simulink model "dynamicANN"  (R2019b)
settings: Solver=VariableStepAuto  StartTime=0.0  StopTime=5  RelTol=1e-3
values from neighbouring files (symbols this model uses):
  a = 87.548e-3    (= 0.087548)    [main.m]
  b = 132.452e-3    (= 0.132452)    [main.m]
  d = 22.452e-3    (= 0.022452)    [main.m]
  delta = [dX 0 0 0; -dX 0 0 0; 0 dXdot 0 0; 0 -dXdot 0 0; 0 0 dY 0; 0 0 -dY 0; 0 0 0 dYdot; 0 0 0 -dYdot]    [dyn_coeff.m]    (also in main.m = 2.5e-05)
  F1 = mass*g-F2    (= 22.4020462598)    [main.m]
  F2 = a*mass*g/(a+b)    (= 14.8072837402)    [main.m]
  g = 9.8    [EOM.m]    (also in main.m = 9.81)
  Jd = 0.047331604    [main.m]
  Jp = 0.00075    [main.m]
  Kps = (Vmax-Vmin)/(Hmax-Hmin)    (= 1666.66666667)    [main.m]
  Ksv = 30    [main.m]
  mass = 3.793    [main.m]
  omega = operational_parameters(1)*2*pi/60    [CalculateLoadCapacity.m]    (also in main.m = 146.607657168)
  s = 30e-3    (= 0.03)    [main.m]    (also in nntrainingsetgen.m = size(XC))
  tau = 0.12    [main.m]
  taus = 0.00125    [main.m]
  Ts = 1/fs    (= 0.001)    [main.m]
libraries: neural x424, simulink x2
(part 1 of 10)
settings Model: Creator=Alexander  LastModifiedBy=Alexander

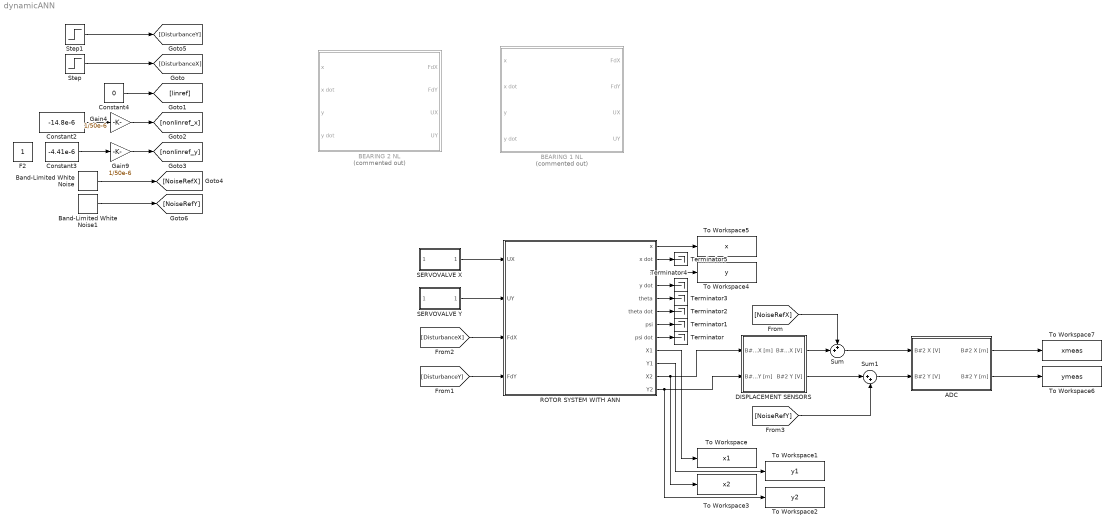
== system dynamicANN ==
  ADC : Subsystem
  BEARING 1 NL : Subsystem  Commented=on
  BEARING 2 NL : Subsystem  Commented=on
  Band-Limited White Noise : simulink/Sources/Band-Limited White Noise  Cov=n_pow  Ts=Ts  seed=[23341]
  Band-Limited White Noise1 : simulink/Sources/Band-Limited White Noise  Cov=n_pow  Ts=1.1*Ts  seed=[23341]
  Constant2 : Constant  Value=-14.8e-6
  Constant3 : Constant  Value=-4.41e-6
  Constant4 : Constant  Value=0
  DISPLACEMENT SENSORS : Subsystem
  Gain4 : Gain  Gain=1/50e-6
  Gain9 : Gain  Gain=1/50e-6
  ROTOR SYSTEM WITH ANN : Subsystem
  SERVOVALVE X : Subsystem
  SERVOVALVE Y : Subsystem
  Step : Step  After=-15  SampleTime=0
  Step1 : Step  After=-15  SampleTime=0
  Sum : Sum  Inputs=++|
  Sum1 : Sum  Inputs=|++
  Terminator{,1..5} (6 alike) : Terminator
  To Workspace : ToWorkspace  VariableName=x1  SampleTime=-1
      settings: Save2DSignal=2-D array (concatenate along first dimension)
  To Workspace1 : ToWorkspace  VariableName=y1  SampleTime=-1
      settings: Save2DSignal=2-D array (concatenate along first dimension)
  To Workspace2 : ToWorkspace  VariableName=y2  SampleTime=-1
      settings: Save2DSignal=2-D array (concatenate along first dimension)
  To Workspace3 : ToWorkspace  VariableName=x2  SampleTime=-1
      settings: Save2DSignal=2-D array (concatenate along first dimension)
  To Workspace4 : ToWorkspace  VariableName=y  SampleTime=-1
      settings: Save2DSignal=2-D array (concatenate along first dimension)
  To Workspace5 : ToWorkspace  VariableName=x  SampleTime=-1
      settings: Save2DSignal=2-D array (concatenate along first dimension)
  To Workspace6 : ToWorkspace  VariableName=ymeas  SampleTime=-1
      settings: Save2DSignal=2-D array (concatenate along first dimension)
  To Workspace7 : ToWorkspace  VariableName=xmeas  SampleTime=-1
      settings: Save2DSignal=2-D array (concatenate along first dimension)
  F2 : Constant  IOType=siggen
  wires:
  ROTOR SYSTEM WITH ANN/10(Y1) -> To Workspace1/1
  ROTOR SYSTEM WITH ANN/9(X1) -> To Workspace/1
  ROTOR SYSTEM WITH ANN/8(psi dot) -> Terminator/1
  ROTOR SYSTEM WITH ANN/6("theta dot ") -> Terminator2/1
  ROTOR SYSTEM WITH ANN/7(psi) -> Terminator1/1
  ROTOR SYSTEM WITH ANN/4(y dot) -> Terminator4/1
  ROTOR SYSTEM WITH ANN/5(theta) -> Terminator3/1
  ROTOR SYSTEM WITH ANN/2(x dot) -> Terminator5/1
  ROTOR SYSTEM WITH ANN/3(y) -> To Workspace4/1
  ROTOR SYSTEM WITH ANN/1("x ") -> To Workspace5/1
  SERVOVALVE Y/1(Uf [F]) -> ROTOR SYSTEM WITH ANN/2(UY)
  SERVOVALVE X/1(Uf [F]) -> ROTOR SYSTEM WITH ANN/1(UX)
  Constant3/1 -> Gain9/1
  Step1/1 -> [DisturbanceY]
  Gain9/1 -> [nonlinref_y]
  Constant2/1 -> Gain4/1
  Constant4/1 -> [linref]
  Step/1 -> [DisturbanceX]
  Gain4/1 -> [nonlinref_x]
  [DisturbanceY] -> ROTOR SYSTEM WITH ANN/4(FdY)
  [DisturbanceX] -> ROTOR SYSTEM WITH ANN/3(FdX)
  Band-Limited White Noise/1 -> [NoiseRefX]
  Band-Limited White Noise1/1 -> [NoiseRefY]
  [NoiseRefY] -> Sum1/2
  Sum/1 -> ADC/1(B#2 X [V])
  Sum1/1 -> ADC/2(B#2 Y [V])
  ADC/2(B#2 Y [m]) -> To Workspace6/1
  ADC/1(B#2 X [m]) -> To Workspace7/1
  ROTOR SYSTEM WITH ANN/12(Y2) -> To Workspace2/1, DISPLACEMENT SENSORS/2(B#2 Y [m])
  ROTOR SYSTEM WITH ANN/11("X2 ") -> To Workspace3/1, DISPLACEMENT SENSORS/1(B#2 X [m])
  DISPLACEMENT SENSORS/1(B#2 X [V]) -> Sum/2
  DISPLACEMENT SENSORS/2(B#2 Y [V]) -> Sum1/1
  [NoiseRefX] -> Sum/1

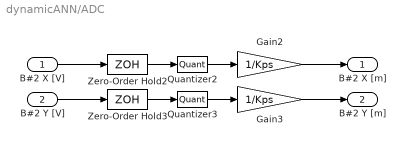
== system dynamicANN/ADC ==
  B#2 X [V] : Inport
  B#2 Y [V] : Inport  Port=2
  Gain2 : Gain  Gain=1/Kps
  Gain3 : Gain  Gain=1/Kps
  Quantizer2 : Quantizer  QuantizationInterval=0.000152587890625
  Quantizer3 : Quantizer  QuantizationInterval=0.000152587890625
  Zero-Order Hold2 : ZeroOrderHold  SampleTime=Ts
  Zero-Order Hold3 : ZeroOrderHold  SampleTime=Ts
  B#2 X [m] : Outport
  B#2 Y [m] : Outport  Port=2
  wires:
  Quantizer2/1 -> Gain2/1
  Quantizer3/1 -> Gain3/1
  B#2 X [V]/1 -> Zero-Order Hold2/1
  Gain2/1 -> B#2 X [m]/1
  Zero-Order Hold2/1 -> Quantizer2/1
  Gain3/1 -> B#2 Y [m]/1
  Zero-Order Hold3/1 -> Quantizer3/1
  B#2 Y [V]/1 -> Zero-Order Hold3/1

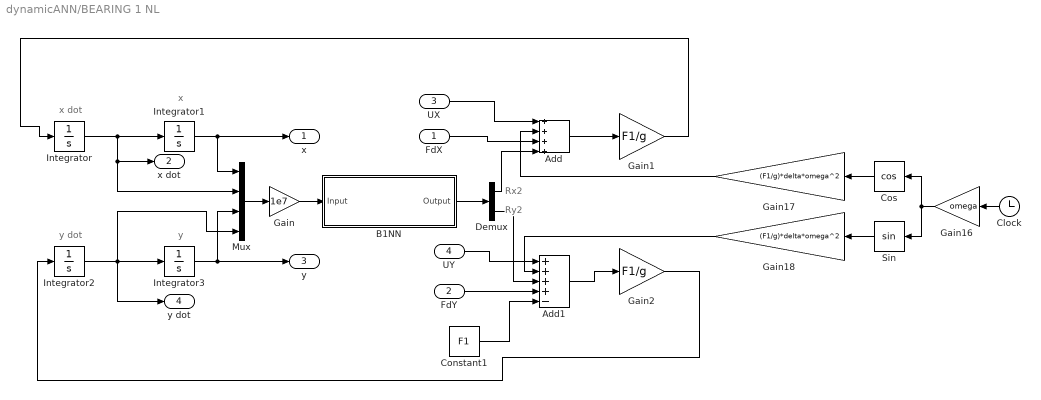
== system dynamicANN/BEARING 1 NL ==
  note: y
  note: x dot
  note: y dot
  note: Rx2
  note: Ry2
  note: x
  FdX : Inport
  FdY : Inport  Port=2
  UX : Inport  Port=3
  UY : Inport  Port=4
  Add : Sum  Inputs=++++
  Add1 : Sum  Inputs=++++-
  B1NN : Subsystem
      mask help: Feed-Forward Neural Network
      mask Display: fprintf('BEARIN #1 NN');port_label('input',1,' X');port_label('output',1,'F');
  Clock : Clock
  Constant1 : Constant  Value=F1
  Cos : Trigonometry  Operator=cos
  Demux : Demux  Outputs=2
  Gain : Gain  Gain=1e7
  Gain1 : Gain  Gain=F1/g
  Gain16 : Gain  Gain=omega
  Gain17 : Gain  Gain=(F1/g)*delta*omega^2
  Gain18 : Gain  Gain=(F1/g)*delta*omega^2
  Gain2 : Gain  Gain=F1/g
  Integrator{,1..3} (4 alike) : Integrator
  Mux : Mux
  Sin : Trigonometry
  x : Outport
  "x dot " : Outport  Port=2
  y : Outport  Port=3
  y dot : Outport  Port=4
  wires:
  Mux/1 -> Gain/1
  B1NN/1(Output) -> Demux/1
  Gain/1 -> B1NN/1(Input)
  Integrator1/1 -> x/1, Mux/1
  Integrator2/1 -> y dot/1, Mux/4, Integrator3/1
  Integrator/1 -> "x dot "/1, Mux/2, Integrator1/1
  Integrator3/1 -> y/1, Mux/3
  Clock/1 -> Gain16/1
  Sin/1 -> Gain18/1
  Cos/1 -> Gain17/1
  Gain2/1 -> Integrator2/1
  Add/1 -> Gain1/1
  Gain16/1 -> Sin/1, Cos/1
  Add1/1 -> Gain2/1
  Gain17/1 -> Add/2
  Gain18/1 -> Add1/2
  Gain1/1 -> Integrator/1
  FdX/1 -> Add/3
  Demux/1 -> Add/4
  FdY/1 -> Add1/4
  Constant1/1 -> Add1/5
  UX/1 -> Add/1
  Demux/2 -> Add1/3
  UY/1 -> Add1/1

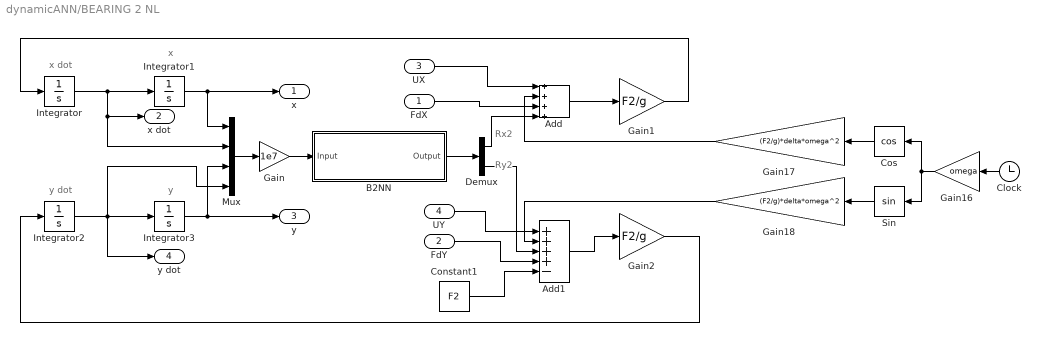
== system dynamicANN/BEARING 2 NL ==
  note: x
  note: x dot
  note: y
  note: y dot
  note: Ry2
  note: Rx2
  FdX : Inport
  FdY : Inport  Port=2
  UX : Inport  Port=3
  UY : Inport  Port=4
  Add : Sum  Inputs=++++
  Add1 : Sum  Inputs=++++-
  B2NN : Subsystem
      mask help: Feed-Forward Neural Network
      mask Display: fprintf('BEARING #2 NN');port_label('input',1,' X');port_label('output',1,'F');
  Clock : Clock
  Constant1 : Constant  Value=F2
  Cos : Trigonometry  Operator=cos
  Demux : Demux  Outputs=2
  Gain : Gain  Gain=1e7
  Gain1 : Gain  Gain=F2/g
  Gain16 : Gain  Gain=omega
  Gain17 : Gain  Gain=(F2/g)*delta*omega^2
  Gain18 : Gain  Gain=(F2/g)*delta*omega^2
  Gain2 : Gain  Gain=F2/g
  Integrator{,1..3} (4 alike) : Integrator
  Mux : Mux
  Sin : Trigonometry
  x : Outport
  "x dot " : Outport  Port=2
  y : Outport  Port=3
  y dot : Outport  Port=4
  wires:
  Add1/1 -> Gain2/1
  Gain1/1 -> Integrator/1
  FdY/1 -> Add1/4
  Integrator/1 -> "x dot "/1, Mux/2, Integrator1/1
  Integrator1/1 -> x/1, Mux/1
  Integrator2/1 -> y dot/1, Mux/4, Integrator3/1
  Add/1 -> Gain1/1
  Integrator3/1 -> y/1, Mux/3
  FdX/1 -> Add/3
  Mux/1 -> Gain/1
  Demux/2 -> Add1/3
  Gain/1 -> B2NN/1(Input)
  Demux/1 -> Add/4
  Gain2/1 -> Integrator2/1
  Constant1/1 -> Add1/5
  B2NN/1(Output) -> Demux/1
  Sin/1 -> Gain18/1
  Cos/1 -> Gain17/1
  Gain16/1 -> Sin/1, Cos/1
  Clock/1 -> Gain16/1
  Gain17/1 -> Add/2
  Gain18/1 -> Add1/2
  UX/1 -> Add/1
  UY/1 -> Add1/1

== system dynamicANN/DISPLACEMENT SENSORS ==
  B#2 X [m] : Inport
  B#2 Y [m] : Inport  Port=2
  Transfer Fcn2 : TransferFcn  Numerator=[Kps]  Denominator=[taus 1]
  Transfer Fcn3 : TransferFcn  Numerator=[Kps]  Denominator=[taus 1]
  B#2 X [V] : Outport
  B#2 Y [V] : Outport  Port=2
  wires:
  B#2 Y [m]/1 -> Transfer Fcn3/1
  B#2 X [m]/1 -> Transfer Fcn2/1
  Transfer Fcn2/1 -> B#2 X [V]/1
  Transfer Fcn3/1 -> B#2 Y [V]/1

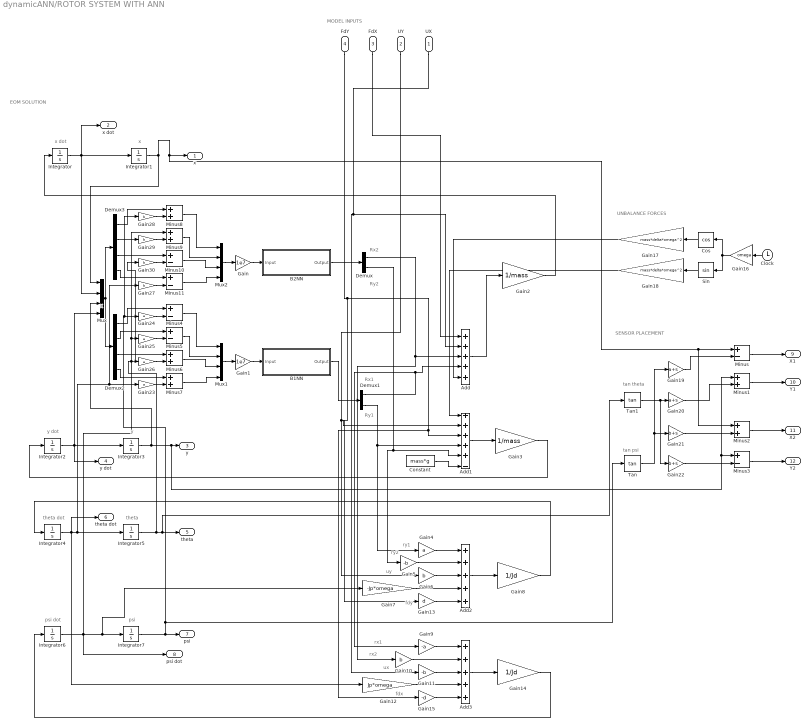
== system dynamicANN/ROTOR SYSTEM WITH ANN ==
  note: SENSOR PLACEMENT
  note: tan theta
  note: EOM SOLUTION
  note: MODEL INPUTS
  note: UNBALANCE FORCES
  note: fdx
  note: ux
  note: rx2
  note: rx1
  note: fdy
  note: uy
  note: ry2
  note: ry1
  note: Ry2
  note: Rx2
  note: X
  note: x dot
  note: x
  note: y
  note: y dot
  note: Ry1
  note: Rx1
  note: theta dot
  note: theta
  note: psi dot
  note: psi
  note: tan psi
  UX : Inport
  UY : Inport  Port=2
  FdX : Inport  Port=3
  FdY : Inport  Port=4
  Add : Sum  Inputs=+++++
  Add1 : Sum  Inputs=+++++-
  Add2 : Sum  Inputs=+++++
  Add3 : Sum  Inputs=+++++
  B1NN : Subsystem
      mask help: Feed-Forward Neural Network
      mask Display: fprintf('BEARIN #1 NN');port_label('input',1,' X');port_label('output',1,'F');
  B2NN : Subsystem
      mask help: Feed-Forward Neural Network
      mask Display: fprintf('BEARING #2 NN');port_label('input',1,' X');port_label('output',1,'F');
  Clock : Clock
  Constant : Constant  Value=mass*g
  Cos : Trigonometry  Operator=cos
  Demux : Demux  Outputs=2
  Demux1 : Demux  Outputs=2
  Demux2 : Demux
  Demux3 : Demux
  Gain : Gain  Gain=1e7
  Gain1 : Gain  Gain=1e7
  Gain{6,10,27..30} (6 alike) : Gain  Gain=b
  Gain11 : Gain  Gain=-b
  Gain12 : Gain  Gain=Jp*omega
  Gain13 : Gain  Gain=d
  Gain14 : Gain  Gain=1/Jd
  Gain15 : Gain  Gain=-d
  Gain16 : Gain  Gain=omega
  Gain17 : Gain  Gain=mass*delta*omega^2
  Gain18 : Gain  Gain=mass*delta*omega^2
  Gain19 : Gain  Gain=a+s
  Gain2 : Gain  Gain=1/mass
  Gain20 : Gain  Gain=a+s
  Gain21 : Gain  Gain=b+s
  Gain22 : Gain  Gain=b+s
  Gain{4,23..26} (5 alike) : Gain  Gain=a
  Gain3 : Gain  Gain=1/mass
  Gain5 : Gain  Gain=-b
  Gain7 : Gain  Gain=-Jp*omega
  Gain8 : Gain  Gain=1/Jd
  Gain9 : Gain  Gain=-a
  Integrator{,1..7} (8 alike) : Integrator
  Minus{,3..5,10..11} (6 alike) : Sum  Inputs=+-
  Minus{1..2,6..9} (6 alike) : Sum
  Mux : Mux
  Mux1 : Mux
  Mux2 : Mux
  Sin : Trigonometry
  Tan : Trigonometry  Operator=tan
  Tan1 : Trigonometry  Operator=tan
  "x " : Outport
  x dot : Outport  Port=2
  y : Outport  Port=3
  y dot : Outport  Port=4
  theta : Outport  Port=5
  "theta dot " : Outport  Port=6
  psi : Outport  Port=7
  psi dot : Outport  Port=8
  X1 : Outport  Port=9
  Y1 : Outport  Port=10
  "X2 " : Outport  Port=11
  Y2 : Outport  Port=12
  wires:
  FdY/1 -> Gain15/1, Add1/3, Gain13/1
  Integrator2/1 -> Mux/4, y dot/1, Integrator3/1
  Integrator3/1 -> Minus1/1, Minus3/1, y/1, Mux/3
  Integrator4/1 -> Gain23/1, Gain27/1, Integrator5/1, Gain12/1, "theta dot "/1
  Integrator6/1 -> psi dot/1, Gain7/1, Integrator7/1, Gain29/1, Gain25/1
  Mux/1 -> Demux2/1, Demux3/1
  Add3/1 -> Gain14/1
  UX/1 -> Gain11/1, Add/2
  Add/1 -> Gain2/1
  Demux1/2 -> Gain4/1, Add1/4
  Gain15/1 -> Add3/5
  Integrator/1 -> x dot/1, Mux/2, Integrator1/1
  Demux/1 -> Gain10/1, Add/3
  UY/1 -> Add1/2, Gain6/1
  Integrator7/1 -> Gain24/1, Gain28/1, Tan/1, psi/1
  Gain/1 -> B2NN/1(Input)
  Gain11/1 -> Add3/3
  Gain12/1 -> Add3/4
  Gain6/1 -> Add2/3
  Gain10/1 -> Add3/2
  Gain9/1 -> Add3/1
  Demux/2 -> Gain5/1, Add1/5
  Add1/1 -> Gain3/1
  B1NN/1(Output) -> Demux1/1
  Gain8/1 -> Integrator4/1
  Integrator1/1 -> "x "/1, Minus2/1, Minus/1, Mux/1
  FdX/1 -> Add/1
  Demux1/1 -> Gain9/1, Add/4
  Add2/1 -> Gain8/1
  B2NN/1(Output) -> Demux/1
  Gain13/1 -> Add2/5
  Gain1/1 -> B1NN/1(Input)
  Gain3/1 -> Integrator2/1
  Gain4/1 -> Add2/1
  Gain7/1 -> Add2/4
  Gain5/1 -> Add2/2
  Gain14/1 -> Integrator6/1
  Gain2/1 -> Integrator/1
  Integrator5/1 -> Gain30/1, Gain26/1, Tan1/1, theta/1
  Constant/1 -> Add1/6
  Clock/1 -> Gain16/1
  Gain16/1 -> Sin/1, Cos/1
  Cos/1 -> Gain17/1
  Sin/1 -> Gain18/1
  Gain17/1 -> Add/5
  Gain18/1 -> Add1/1
  Gain19/1 -> Minus/2
  Tan/1 -> Gain19/1, Gain21/1
  Minus/1 -> X1/1
  Tan1/1 -> Gain22/1, Gain20/1
  Gain20/1 -> Minus1/2
  Minus1/1 -> Y1/1
  Gain21/1 -> Minus2/2
  Minus2/1 -> "X2 "/1
  Minus3/1 -> Y2/1
  Gain22/1 -> Minus3/2
  Mux1/1 -> Gain1/1
  Minus4/1 -> Mux1/1
  Minus5/1 -> Mux1/2
  Minus7/1 -> Mux1/4
  Minus6/1 -> Mux1/3
  Gain24/1 -> Minus4/2
  Gain25/1 -> Minus5/2
  Gain23/1 -> Minus7/2
  Demux2/1 -> Minus4/1
  Demux2/2 -> Minus5/1
  Demux2/3 -> Minus6/1
  Gain26/1 -> Minus6/2
  Demux2/4 -> Minus7/1
  Gain29/1 -> Minus9/2
  Gain28/1 -> Minus8/2
  Minus8/1 -> Mux2/1
  Gain30/1 -> Minus10/2
  Demux3/3 -> Minus10/1
  Minus10/1 -> Mux2/3
  Demux3/2 -> Minus9/1
  Demux3/4 -> Minus11/1
  Demux3/1 -> Minus8/1
  Minus9/1 -> Mux2/2
  Gain27/1 -> Minus11/2
  Mux2/1 -> Gain/1
  Minus11/1 -> Mux2/4

== system dynamicANN/SERVOVALVE X ==
  Uv [V] : Inport
  Transfer Fcn : TransferFcn  Numerator=Ksv  Denominator=[tau 1]
  Uf [F] : Outport
  wires:
  Transfer Fcn/1 -> Uf [F]/1
  Uv [V]/1 -> Transfer Fcn/1

== system dynamicANN/SERVOVALVE Y ==
  Uv [V] : Inport
  Transfer Fcn : TransferFcn  Numerator=Ksv  Denominator=[tau 1]
  Uf [F] : Outport
  wires:
  Uv [V]/1 -> Transfer Fcn/1
  Transfer Fcn/1 -> Uf [F]/1

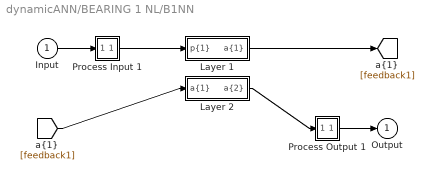
== system dynamicANN/BEARING 1 NL/B1NN ==
  Input : Inport  PortDimensions=4
      mask Display: e = 0.06;c1 = [120 230 180]/255;c2 = ([120 230 180]+0)/(256+128);c3 = ([120 230 180]+128)/(256+128);patch([0 1 1 0],[0 0 1 1],c1);patch([0 1 1 1-e 1-e 0+e],[0 0 1 1-e 0+e 0+e],c2);patch([0 0 1 1-e 0+e 0+e],[0 1 1 1-e 1-e 0+e],c3);plot([0 1 1 0 0],[0 0 1 1 0]);
  Layer 1 : Subsystem
      mask Display: e = 0.06;c1 = [120 150 230]/255;c2 = ([120 150 230]+0)/383;c3 = ([120 150 230]+128)/383;patch([0 1 1 0],[0 0 1 1],c1);patch([0 1 1 1-e 1-e 0+e],[0 0 1 1-e 0+e 0+e],c2);patch([0 0 1 1-e 0+e 0+e],[0 1 1 1-e 1-e 0+e],c3);plot([0 1 1 0 0],[0 0 1 1 0]);
  Layer 2 : Subsystem
      mask Display: e = 0.06;c1 = [120 150 230]/255;c2 = ([120 150 230]+0)/383;c3 = ([120 150 230]+128)/383;patch([0 1 1 0],[0 0 1 1],c1);patch([0 1 1 1-e 1-e 0+e],[0 0 1 1-e 0+e 0+e],c2);patch([0 0 1 1-e 0+e 0+e],[0 1 1 1-e 1-e 0+e],c3);plot([0 1 1 0 0],[0 0 1 1 0]);
  Process Input 1 : Subsystem
      mask Display: e = 0.06;c1 = [120 150 230]/255;c2 = ([120 150 230]+0)/383;c3 = ([120 150 230]+128)/383;patch([0 1 1 0],[0 0 1 1],c1);patch([0 1 1 1-e 1-e 0+e],[0 0 1 1-e 0+e 0+e],c2);patch([0 0 1 1-e 0+e 0+e],[0 1 1 1-e 1-e 0+e],c3);plot([0 1 1 0 0],[0 0 1 1 0]);
  Process Output 1 : Subsystem
      mask Display: e = 0.06;c1 = [120 150 230]/255;c2 = ([120 150 230]+0)/383;c3 = ([120 150 230]+128)/383;patch([0 1 1 0],[0 0 1 1],c1);patch([0 1 1 1-e 1-e 0+e],[0 0 1 1-e 0+e 0+e],c2);patch([0 0 1 1-e 0+e 0+e],[0 1 1 1-e 1-e 0+e],c3);plot([0 1 1 0 0],[0 0 1 1 0]);
  Output : Outport  InitialOutput=[0;0]
      mask Display: e = 0.06;c1 = [120 230 180]/255;c2 = ([120 230 180]+0)/(256+128);c3 = ([120 230 180]+128)/(256+128);patch([0 1 1 0],[0 0 1 1],c1);patch([0 1 1 1-e 1-e 0+e],[0 0 1 1-e 0+e 0+e],c2);patch([0 0 1 1-e 0+e 0+e],[0 1 1 1-e 1-e 0+e],c3);plot([0 1 1 0 0],[0 0 1 1 0]);
  wires:
  Input/1 -> Process Input 1/1(x)
  Process Output 1/1(y) -> Output/1
  Process Input 1/1(p) -> Layer 1/1("p{1}")
  Layer 1/1("a{1}") -> [feedback1]
  [feedback1] -> Layer 2/1("a{1} ")
  Layer 2/1("a{2}") -> Process Output 1/1(a)

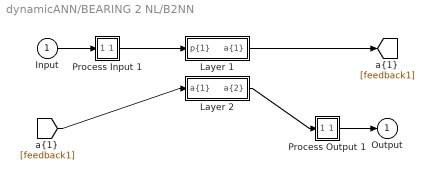
== system dynamicANN/BEARING 2 NL/B2NN ==
  Input : Inport  PortDimensions=4
      mask Display: e = 0.06;c1 = [120 230 180]/255;c2 = ([120 230 180]+0)/(256+128);c3 = ([120 230 180]+128)/(256+128);patch([0 1 1 0],[0 0 1 1],c1);patch([0 1 1 1-e 1-e 0+e],[0 0 1 1-e 0+e 0+e],c2);patch([0 0 1 1-e 0+e 0+e],[0 1 1 1-e 1-e 0+e],c3);plot([0 1 1 0 0],[0 0 1 1 0]);
  Layer 1 : Subsystem
      mask Display: e = 0.06;c1 = [120 150 230]/255;c2 = ([120 150 230]+0)/383;c3 = ([120 150 230]+128)/383;patch([0 1 1 0],[0 0 1 1],c1);patch([0 1 1 1-e 1-e 0+e],[0 0 1 1-e 0+e 0+e],c2);patch([0 0 1 1-e 0+e 0+e],[0 1 1 1-e 1-e 0+e],c3);plot([0 1 1 0 0],[0 0 1 1 0]);
  Layer 2 : Subsystem
      mask Display: e = 0.06;c1 = [120 150 230]/255;c2 = ([120 150 230]+0)/383;c3 = ([120 150 230]+128)/383;patch([0 1 1 0],[0 0 1 1],c1);patch([0 1 1 1-e 1-e 0+e],[0 0 1 1-e 0+e 0+e],c2);patch([0 0 1 1-e 0+e 0+e],[0 1 1 1-e 1-e 0+e],c3);plot([0 1 1 0 0],[0 0 1 1 0]);
  Process Input 1 : Subsystem
      mask Display: e = 0.06;c1 = [120 150 230]/255;c2 = ([120 150 230]+0)/383;c3 = ([120 150 230]+128)/383;patch([0 1 1 0],[0 0 1 1],c1);patch([0 1 1 1-e 1-e 0+e],[0 0 1 1-e 0+e 0+e],c2);patch([0 0 1 1-e 0+e 0+e],[0 1 1 1-e 1-e 0+e],c3);plot([0 1 1 0 0],[0 0 1 1 0]);
  Process Output 1 : Subsystem
      mask Display: e = 0.06;c1 = [120 150 230]/255;c2 = ([120 150 230]+0)/383;c3 = ([120 150 230]+128)/383;patch([0 1 1 0],[0 0 1 1],c1);patch([0 1 1 1-e 1-e 0+e],[0 0 1 1-e 0+e 0+e],c2);patch([0 0 1 1-e 0+e 0+e],[0 1 1 1-e 1-e 0+e],c3);plot([0 1 1 0 0],[0 0 1 1 0]);
  Output : Outport  InitialOutput=[0;0]
      mask Display: e = 0.06;c1 = [120 230 180]/255;c2 = ([120 230 180]+0)/(256+128);c3 = ([120 230 180]+128)/(256+128);patch([0 1 1 0],[0 0 1 1],c1);patch([0 1 1 1-e 1-e 0+e],[0 0 1 1-e 0+e 0+e],c2);patch([0 0 1 1-e 0+e 0+e],[0 1 1 1-e 1-e 0+e],c3);plot([0 1 1 0 0],[0 0 1 1 0]);
  wires:
  Input/1 -> Process Input 1/1(x)
  Process Output 1/1(y) -> Output/1
  Process Input 1/1(p) -> Layer 1/1("p{1}")
  Layer 1/1("a{1}") -> [feedback1]
  [feedback1] -> Layer 2/1("a{1} ")
  Layer 2/1("a{2}") -> Process Output 1/1(a)

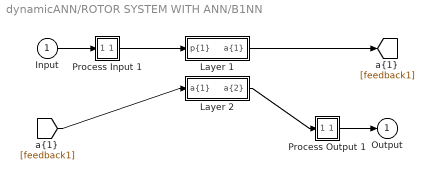
== system dynamicANN/ROTOR SYSTEM WITH ANN/B1NN ==
  Input : Inport  PortDimensions=4
      mask Display: e = 0.06;c1 = [120 230 180]/255;c2 = ([120 230 180]+0)/(256+128);c3 = ([120 230 180]+128)/(256+128);patch([0 1 1 0],[0 0 1 1],c1);patch([0 1 1 1-e 1-e 0+e],[0 0 1 1-e 0+e 0+e],c2);patch([0 0 1 1-e 0+e 0+e],[0 1 1 1-e 1-e 0+e],c3);plot([0 1 1 0 0],[0 0 1 1 0]);
  Layer 1 : Subsystem
      mask Display: e = 0.06;c1 = [120 150 230]/255;c2 = ([120 150 230]+0)/383;c3 = ([120 150 230]+128)/383;patch([0 1 1 0],[0 0 1 1],c1);patch([0 1 1 1-e 1-e 0+e],[0 0 1 1-e 0+e 0+e],c2);patch([0 0 1 1-e 0+e 0+e],[0 1 1 1-e 1-e 0+e],c3);plot([0 1 1 0 0],[0 0 1 1 0]);
  Layer 2 : Subsystem
      mask Display: e = 0.06;c1 = [120 150 230]/255;c2 = ([120 150 230]+0)/383;c3 = ([120 150 230]+128)/383;patch([0 1 1 0],[0 0 1 1],c1);patch([0 1 1 1-e 1-e 0+e],[0 0 1 1-e 0+e 0+e],c2);patch([0 0 1 1-e 0+e 0+e],[0 1 1 1-e 1-e 0+e],c3);plot([0 1 1 0 0],[0 0 1 1 0]);
  Process Input 1 : Subsystem
      mask Display: e = 0.06;c1 = [120 150 230]/255;c2 = ([120 150 230]+0)/383;c3 = ([120 150 230]+128)/383;patch([0 1 1 0],[0 0 1 1],c1);patch([0 1 1 1-e 1-e 0+e],[0 0 1 1-e 0+e 0+e],c2);patch([0 0 1 1-e 0+e 0+e],[0 1 1 1-e 1-e 0+e],c3);plot([0 1 1 0 0],[0 0 1 1 0]);
  Process Output 1 : Subsystem
      mask Display: e = 0.06;c1 = [120 150 230]/255;c2 = ([120 150 230]+0)/383;c3 = ([120 150 230]+128)/383;patch([0 1 1 0],[0 0 1 1],c1);patch([0 1 1 1-e 1-e 0+e],[0 0 1 1-e 0+e 0+e],c2);patch([0 0 1 1-e 0+e 0+e],[0 1 1 1-e 1-e 0+e],c3);plot([0 1 1 0 0],[0 0 1 1 0]);
  Output : Outport  InitialOutput=[0;0]
      mask Display: e = 0.06;c1 = [120 230 180]/255;c2 = ([120 230 180]+0)/(256+128);c3 = ([120 230 180]+128)/(256+128);patch([0 1 1 0],[0 0 1 1],c1);patch([0 1 1 1-e 1-e 0+e],[0 0 1 1-e 0+e 0+e],c2);patch([0 0 1 1-e 0+e 0+e],[0 1 1 1-e 1-e 0+e],c3);plot([0 1 1 0 0],[0 0 1 1 0]);
  wires:
  Input/1 -> Process Input 1/1(x)
  Process Output 1/1(y) -> Output/1
  Process Input 1/1(p) -> Layer 1/1("p{1}")
  Layer 1/1("a{1}") -> [feedback1]
  [feedback1] -> Layer 2/1("a{1} ")
  Layer 2/1("a{2}") -> Process Output 1/1(a)

== system dynamicANN/ROTOR SYSTEM WITH ANN/B2NN ==
  Input : Inport  PortDimensions=4
      mask Display: e = 0.06;c1 = [120 230 180]/255;c2 = ([120 230 180]+0)/(256+128);c3 = ([120 230 180]+128)/(256+128);patch([0 1 1 0],[0 0 1 1],c1);patch([0 1 1 1-e 1-e 0+e],[0 0 1 1-e 0+e 0+e],c2);patch([0 0 1 1-e 0+e 0+e],[0 1 1 1-e 1-e 0+e],c3);plot([0 1 1 0 0],[0 0 1 1 0]);
  Layer 1 : Subsystem
      mask Display: e = 0.06;c1 = [120 150 230]/255;c2 = ([120 150 230]+0)/383;c3 = ([120 150 230]+128)/383;patch([0 1 1 0],[0 0 1 1],c1);patch([0 1 1 1-e 1-e 0+e],[0 0 1 1-e 0+e 0+e],c2);patch([0 0 1 1-e 0+e 0+e],[0 1 1 1-e 1-e 0+e],c3);plot([0 1 1 0 0],[0 0 1 1 0]);
  Layer 2 : Subsystem
      mask Display: e = 0.06;c1 = [120 150 230]/255;c2 = ([120 150 230]+0)/383;c3 = ([120 150 230]+128)/383;patch([0 1 1 0],[0 0 1 1],c1);patch([0 1 1 1-e 1-e 0+e],[0 0 1 1-e 0+e 0+e],c2);patch([0 0 1 1-e 0+e 0+e],[0 1 1 1-e 1-e 0+e],c3);plot([0 1 1 0 0],[0 0 1 1 0]);
  Process Input 1 : Subsystem
      mask Display: e = 0.06;c1 = [120 150 230]/255;c2 = ([120 150 230]+0)/383;c3 = ([120 150 230]+128)/383;patch([0 1 1 0],[0 0 1 1],c1);patch([0 1 1 1-e 1-e 0+e],[0 0 1 1-e 0+e 0+e],c2);patch([0 0 1 1-e 0+e 0+e],[0 1 1 1-e 1-e 0+e],c3);plot([0 1 1 0 0],[0 0 1 1 0]);
  Process Output 1 : Subsystem
      mask Display: e = 0.06;c1 = [120 150 230]/255;c2 = ([120 150 230]+0)/383;c3 = ([120 150 230]+128)/383;patch([0 1 1 0],[0 0 1 1],c1);patch([0 1 1 1-e 1-e 0+e],[0 0 1 1-e 0+e 0+e],c2);patch([0 0 1 1-e 0+e 0+e],[0 1 1 1-e 1-e 0+e],c3);plot([0 1 1 0 0],[0 0 1 1 0]);
  Output : Outport  InitialOutput=[0;0]
      mask Display: e = 0.06;c1 = [120 230 180]/255;c2 = ([120 230 180]+0)/(256+128);c3 = ([120 230 180]+128)/(256+128);patch([0 1 1 0],[0 0 1 1],c1);patch([0 1 1 1-e 1-e 0+e],[0 0 1 1-e 0+e 0+e],c2);patch([0 0 1 1-e 0+e 0+e],[0 1 1 1-e 1-e 0+e],c3);plot([0 1 1 0 0],[0 0 1 1 0]);
  wires:
  Input/1 -> Process Input 1/1(x)
  Process Output 1/1(y) -> Output/1
  Process Input 1/1(p) -> Layer 1/1("p{1}")
  Layer 1/1("a{1}") -> [feedback1]
  [feedback1] -> Layer 2/1("a{1} ")
  Layer 2/1("a{2}") -> Process Output 1/1(a)

== system dynamicANN/BEARING 1 NL/B1NN/Layer 1 ==
  "p{1}" : Inport  PortDimensions=4
      mask Display: e = 0.06;c1 = [120 230 180]/255;c2 = ([120 230 180]+0)/(256+128);c3 = ([120 230 180]+128)/(256+128);patch([0 1 1 0],[0 0 1 1],c1);patch([0 1 1 1-e 1-e 0+e],[0 0 1 1-e 0+e 0+e],c2);patch([0 0 1 1-e 0+e 0+e],[0 1 1 1-e 1-e 0+e],c3);plot([0 1 1 0 0],[0 0 1 1 0]);
  Delays 1 : Subsystem
      mask Display: e = 0.06;c1 = [120 150 230]/255;c2 = ([120 150 230]+0)/383;c3 = ([120 150 230]+128)/383;patch([0 1 1 0],[0 0 1 1],c1);patch([0 1 1 1-e 1-e 0+e],[0 0 1 1-e 0+e 0+e],c2);patch([0 0 1 1-e 0+e 0+e],[0 1 1 1-e 1-e 0+e],c3);plot([0 1 1 0 0],[0 0 1 1 0]);disp('0');
  "IW{1,1}" : Subsystem
      mask Display: e = 0.06;c1 = [120 150 230]/255;c2 = ([120 150 230]+0)/383;c3 = ([120 150 230]+128)/383;patch([0 1 1 0],[0 0 1 1],c1);patch([0 1 1 1-e 1-e 0+e],[0 0 1 1-e 0+e 0+e],c2);patch([0 0 1 1-e 0+e 0+e],[0 1 1 1-e 1-e 0+e],c3);plot([0 1 1 0 0],[0 0 1 1 0]);disp('W');
  "b{1}" : Constant  Value=[0.181633277786767910466636521960026584565639495849609375;0.070875904756337371193097851573838852345943450927734375;-1.24719754114895220453718138742260634899139404296875;0.349807597905259337611738601481192745268344879150390625;-2.257395498018872626033726191963069140911102294921875;0.56411301204936570297121534167672507464885711669921875;-1.0623076449073216576124423227156512439250946044921875;1.3261277037602827721940457195159979164600372314453125;1.6348260834900951721238016034476459026336669921875;1.5138737414120957414098711524275131523609161376953125;0.4020686473945700445398188094259239733219146728515625;1.2524466038126196298918557658907957375049591064453125;3.363853052384917052819446325884200632572174072265625;-0.8830413361956737094971003898535855114459991455078125;4.7786496020530666584136270103044807910919189453125;-4.9577311401354933195761987008154392242431640625;1.888217706423764408185661523020826280117034912109375;0.159845267806201174476399273771676234900951385498046875;-3.803127792976743304365072617656551301479339599609375;-1.99592377305407264742598272277973592281341552734375;-0.58431582957179417636695006876834668219089508056640625;-5.629678072906084906890100683085620403289794921875;2.164562257956847535211863942095078527927398681640625;1.1742110878742557655840528241242282092571258544921875;-1.4613298628920148303222958929836750030517578125;0.88927167428907927249071008191094733774662017822265625;-0.03284845738244450419340836333503830246627330780029296875;5.87363473702414307098251811112277209758758544921875;-5.40481662522351857802505037398077547550201416015625;-7.9743347740786365562826176756061613559722900390625;-4.92172626389882150732546506333164870738983154296875;-2.161011455396362190839454342494718730449676513671875;-5.06722690094917549430419967393390834331512451171875;-5.3287305224634309297471190802752971649169921875;-0.64630765275112544987479168412392027676105499267578125;0.66714709685646400583181048205005936324596405029296875;4.93233697003778548406671689008362591266632080078125;-1.732977582639430469413355240249074995517730712890625;-1.908681806352313881092186420573852956295013427734375;2.01843370502494234841606157715432345867156982421875;5.233844820546135423455780255608260631561279296875;-1.214541408329711469349376784521155059337615966796875;1.9876238893938953378182077358360402286052703857421875;0.06721918587072427120343576234517968259751796722412109375;0.76141795842792869830617519255611114203929901123046875;-4.0025443828292512904454270028509199619293212890625;0.63094205509544487586737204765086062252521514892578125;0.615045803373759358834149679751135408878326416015625;-1.0170568312721484094396373620838858187198638916015625;9.1804013107524031767070482601411640644073486328125;-0.5722890567479497203606797484098933637142181396484375;-5.038267835849712383833320927806198596954345703125;0.419509696131923737194568957420415244996547698974609375;-1.0661316915627254697795933680026791989803314208984375;1.2472196822626464562944192948634736239910125732421875;-0.2200263246403744432644344897198607213795185089111328125;1.630345291318326506058156155631877481937408447265625;0.87107474322196054572486900724470615386962890625;1.2689953165555760694616083128494210541248321533203125;0.681018751916095954612728746724314987659454345703125;2.413082616196982943534976584487594664096832275390625;0.0196006134151332882253893075130690704099833965301513671875;1.33728973082240454317570765851996839046478271484375;-0.39696093317092218111241663791588507592678070068359375;1.5529947289365697571383861941285431385040283203125;0.95926187851158550845553918406949378550052642822265625;-0.004745806788341252503704570386844352469779551029205322265625;0.52096120648883703641018882990465499460697174072265625;2.62011306102542551599299258668906986713409423828125;1.702495991802877473020316756446845829486846923828125;-2.020250840664974401050812957691960036754608154296875;0.03237340384429125694776274713149177841842174530029296875 ...(+1513 chars)]
      mask Display: e = 0.06;c1 = [120 150 230]/255;c2 = ([120 150 230]+0)/383;c3 = ([120 150 230]+128)/383;patch([0 1 1 0],[0 0 1 1],c1);patch([0 1 1 1-e 1-e 0+e],[0 0 1 1-e 0+e 0+e],c2);patch([0 0 1 1-e 0+e 0+e],[0 1 1 1-e 1-e 0+e],c3);plot([0 1 1 0 0],[0 0 1 1 0]);disp('b');
  netsum : Sum  Inputs=2  SaturateOnIntegerOverflow=on  InputSameDT=on  OutDataTypeStr=Inherit: Same as first input
      mask Display: e = 0.06;c1 = [120 150 230]/255;c2 = ([120 150 230]+0)/383;c3 = ([120 150 230]+128)/383;patch([0 1 1 0],[0 0 1 1],c1);patch([0 1 1 1-e 1-e 0+e],[0 0 1 1-e 0+e 0+e],c2);patch([0 0 1 1-e 0+e 0+e],[0 1 1 1-e 1-e 0+e],c3);plot([0 1 1 0 0],[0 0 1 1 0]);disp('+');
  tansig : neural/Transfer Functions/tansig
      settings: SourceProductName=Deep Learning Toolbox
  "a{1}" : Outport  InitialOutput=[0;0;0;0;0;0;0;0;0;0;0;0;0;0;0;0;0;0;0;0;0;0;0;0;0;0;0;0;0;0;0;0;0;0;0;0;0;0;0;0;0;0;0;0;0;0;0;0;0;0;0;0;0;0;0;0;0;0;0;0;0;0;0;0;0;0;0;0;0;0;0;0;0;0;0;0;0;0;0;0;0;0;0;0;0;0;0;0;0;0;0;0;0;0;0;0;0;0;0;0]
      mask Display: e = 0.06;c1 = [120 230 180]/255;c2 = ([120 230 180]+0)/(256+128);c3 = ([120 230 180]+128)/(256+128);patch([0 1 1 0],[0 0 1 1],c1);patch([0 1 1 1-e 1-e 0+e],[0 0 1 1-e 0+e 0+e],c2);patch([0 0 1 1-e 0+e 0+e],[0 1 1 1-e 1-e 0+e],c3);plot([0 1 1 0 0],[0 0 1 1 0]);
  wires:
  "p{1}"/1 -> Delays 1/1("p{1}")
  Delays 1/1("pd{1,1}") -> "IW{1,1}"/1("pd{1,1}")
  "IW{1,1}"/1("iz{1,1}") -> netsum/1
  "b{1}"/1 -> netsum/2
  netsum/1 -> tansig/1
  tansig/1 -> "a{1}"/1

== system dynamicANN/BEARING 1 NL/B1NN/Layer 2 ==
  "a{1} " : Inport  PortDimensions=100
      mask Display: e = 0.06;c1 = [120 230 180]/255;c2 = ([120 230 180]+0)/(256+128);c3 = ([120 230 180]+128)/(256+128);patch([0 1 1 0],[0 0 1 1],c1);patch([0 1 1 1-e 1-e 0+e],[0 0 1 1-e 0+e 0+e],c2);patch([0 0 1 1-e 0+e 0+e],[0 1 1 1-e 1-e 0+e],c3);plot([0 1 1 0 0],[0 0 1 1 0]);
  Delays 1 : Subsystem
      mask Display: e = 0.06;c1 = [120 150 230]/255;c2 = ([120 150 230]+0)/383;c3 = ([120 150 230]+128)/383;patch([0 1 1 0],[0 0 1 1],c1);patch([0 1 1 1-e 1-e 0+e],[0 0 1 1-e 0+e 0+e],c2);patch([0 0 1 1-e 0+e 0+e],[0 1 1 1-e 1-e 0+e],c3);plot([0 1 1 0 0],[0 0 1 1 0]);disp('0');
  "LW{2,1}" : Subsystem
      mask Display: e = 0.06;c1 = [120 150 230]/255;c2 = ([120 150 230]+0)/383;c3 = ([120 150 230]+128)/383;patch([0 1 1 0],[0 0 1 1],c1);patch([0 1 1 1-e 1-e 0+e],[0 0 1 1-e 0+e 0+e],c2);patch([0 0 1 1-e 0+e 0+e],[0 1 1 1-e 1-e 0+e],c3);plot([0 1 1 0 0],[0 0 1 1 0]);disp('W');
  "b{2}" : Constant  Value=[-0.342223457267687714011827893045847304165363311767578125;0.5690036877110060675732938761939294636249542236328125]
      mask Display: e = 0.06;c1 = [120 150 230]/255;c2 = ([120 150 230]+0)/383;c3 = ([120 150 230]+128)/383;patch([0 1 1 0],[0 0 1 1],c1);patch([0 1 1 1-e 1-e 0+e],[0 0 1 1-e 0+e 0+e],c2);patch([0 0 1 1-e 0+e 0+e],[0 1 1 1-e 1-e 0+e],c3);plot([0 1 1 0 0],[0 0 1 1 0]);disp('b');
  netsum : Sum  Inputs=2  SaturateOnIntegerOverflow=on  InputSameDT=on  OutDataTypeStr=Inherit: Same as first input
      mask Display: e = 0.06;c1 = [120 150 230]/255;c2 = ([120 150 230]+0)/383;c3 = ([120 150 230]+128)/383;patch([0 1 1 0],[0 0 1 1],c1);patch([0 1 1 1-e 1-e 0+e],[0 0 1 1-e 0+e 0+e],c2);patch([0 0 1 1-e 0+e 0+e],[0 1 1 1-e 1-e 0+e],c3);plot([0 1 1 0 0],[0 0 1 1 0]);disp('+');
  purelin : neural/Transfer Functions/purelin
      settings: SourceProductName=Deep Learning Toolbox
  "a{2}" : Outport  InitialOutput=[0;0]
      mask Display: e = 0.06;c1 = [120 230 180]/255;c2 = ([120 230 180]+0)/(256+128);c3 = ([120 230 180]+128)/(256+128);patch([0 1 1 0],[0 0 1 1],c1);patch([0 1 1 1-e 1-e 0+e],[0 0 1 1-e 0+e 0+e],c2);patch([0 0 1 1-e 0+e 0+e],[0 1 1 1-e 1-e 0+e],c3);plot([0 1 1 0 0],[0 0 1 1 0]);
  wires:
  "a{1} "/1 -> Delays 1/1("p{2}")
  Delays 1/1("pd{2,1}") -> "LW{2,1}"/1("ad{2,1}")
  "LW{2,1}"/1("lz{2,1}") -> netsum/1
  "b{2}"/1 -> netsum/2
  netsum/1 -> purelin/1
  purelin/1 -> "a{2}"/1

== system dynamicANN/BEARING 1 NL/B1NN/Process Input 1 ==
  x : Inport  PortDimensions=4
      mask Display: e = 0.06;c1 = [120 230 180]/255;c2 = ([120 230 180]+0)/(256+128);c3 = ([120 230 180]+128)/(256+128);patch([0 1 1 0],[0 0 1 1],c1);patch([0 1 1 1-e 1-e 0+e],[0 0 1 1-e 0+e 0+e],c2);patch([0 0 1 1-e 0+e 0+e],[0 1 1 1-e 1-e 0+e],c3);plot([0 1 1 0 0],[0 0 1 1 0]);
  mapminmax : neural/Processing Functions/mapminmax  xmin=[-413.338445747307901001477148384;-74739.7828198331408202648162842;-415.187022501626017856324324384;-89747.7004398032004246488213539]  xmax=[417.586189284466797744244104251;74696.3661857289116596803069115;397.43934373063848397578112781;59322.5202224319145898334681988]  ymin=-1  ymax=1
      settings: SourceProductName=Deep Learning Toolbox
  p : Outport  PortDimensions=4
      mask Display: e = 0.06;c1 = [120 230 180]/255;c2 = ([120 230 180]+0)/(256+128);c3 = ([120 230 180]+128)/(256+128);patch([0 1 1 0],[0 0 1 1],c1);patch([0 1 1 1-e 1-e 0+e],[0 0 1 1-e 0+e 0+e],c2);patch([0 0 1 1-e 0+e 0+e],[0 1 1 1-e 1-e 0+e],c3);plot([0 1 1 0 0],[0 0 1 1 0]);
  wires:
  x/1 -> mapminmax/1
  mapminmax/1 -> p/1

== system dynamicANN/BEARING 1 NL/B1NN/Process Output 1 ==
  a : Inport  PortDimensions=2
      mask Display: e = 0.06;c1 = [120 230 180]/255;c2 = ([120 230 180]+0)/(256+128);c3 = ([120 230 180]+128)/(256+128);patch([0 1 1 0],[0 0 1 1],c1);patch([0 1 1 1-e 1-e 0+e],[0 0 1 1-e 0+e 0+e],c2);patch([0 0 1 1-e 0+e 0+e],[0 1 1 1-e 1-e 0+e],c3);plot([0 1 1 0 0],[0 0 1 1 0]);
  mapminmax_reverse : neural/Processing Functions/mapminmax_reverse  xmin=[-108.739456947512550755163829308;-83.5692461035311708883455139585]  xmax=[107.216624359632618279647431336;132.674050199725030552144744433]  ymin=-1  ymax=1
      settings: SourceProductName=Deep Learning Toolbox
  y : Outport  PortDimensions=2
      mask Display: e = 0.06;c1 = [120 230 180]/255;c2 = ([120 230 180]+0)/(256+128);c3 = ([120 230 180]+128)/(256+128);patch([0 1 1 0],[0 0 1 1],c1);patch([0 1 1 1-e 1-e 0+e],[0 0 1 1-e 0+e 0+e],c2);patch([0 0 1 1-e 0+e 0+e],[0 1 1 1-e 1-e 0+e],c3);plot([0 1 1 0 0],[0 0 1 1 0]);
  wires:
  a/1 -> mapminmax_reverse/1
  mapminmax_reverse/1 -> y/1

== system dynamicANN/BEARING 2 NL/B2NN/Layer 1 ==
  "p{1}" : Inport  PortDimensions=4
      mask Display: e = 0.06;c1 = [120 230 180]/255;c2 = ([120 230 180]+0)/(256+128);c3 = ([120 230 180]+128)/(256+128);patch([0 1 1 0],[0 0 1 1],c1);patch([0 1 1 1-e 1-e 0+e],[0 0 1 1-e 0+e 0+e],c2);patch([0 0 1 1-e 0+e 0+e],[0 1 1 1-e 1-e 0+e],c3);plot([0 1 1 0 0],[0 0 1 1 0]);
  Delays 1 : Subsystem
      mask Display: e = 0.06;c1 = [120 150 230]/255;c2 = ([120 150 230]+0)/383;c3 = ([120 150 230]+128)/383;patch([0 1 1 0],[0 0 1 1],c1);patch([0 1 1 1-e 1-e 0+e],[0 0 1 1-e 0+e 0+e],c2);patch([0 0 1 1-e 0+e 0+e],[0 1 1 1-e 1-e 0+e],c3);plot([0 1 1 0 0],[0 0 1 1 0]);disp('0');
  "IW{1,1}" : Subsystem
      mask Display: e = 0.06;c1 = [120 150 230]/255;c2 = ([120 150 230]+0)/383;c3 = ([120 150 230]+128)/383;patch([0 1 1 0],[0 0 1 1],c1);patch([0 1 1 1-e 1-e 0+e],[0 0 1 1-e 0+e 0+e],c2);patch([0 0 1 1-e 0+e 0+e],[0 1 1 1-e 1-e 0+e],c3);plot([0 1 1 0 0],[0 0 1 1 0]);disp('W');
  "b{1}" : Constant  Value=[0.77364063658353299235415079238009639084339141845703125;-0.5742401500824383386856197830638848245143890380859375;2.18924884343246173301622548024170100688934326171875;0.7247679770582233782505454655620269477367401123046875;1.50920298605198599517507318523712456226348876953125;0.2251254120036607908605930106205050833523273468017578125;1.31581849386470395302239921875298023223876953125;-1.4439178611363931992173093021847307682037353515625;-0.6388738634319419684715057883295230567455291748046875;0.42713022702700664812169861761503852903842926025390625;-5.50585208820272331564638079726137220859527587890625;1.0116121407127753872856601446983404457569122314453125;0.1855740272752877950690475472583784721791744232177734375;-2.752365697458559079535689306794665753841400146484375;-5.11790555901796029303341128979809582233428955078125;-0.338655420078370517078525381293729878962039947509765625;1.1393557433472689677245170969399623572826385498046875;-2.759792246021837147651467603282071650028228759765625;0.397902004749398463534504344352171756327152252197265625;3.409108583987378704449611177551560103893280029296875;0.5735207395663535212548822528333403170108795166015625;6.01140115256299356616409568232484161853790283203125;1.7685521361064504564097887850948609411716461181640625;-0.340503549829671514626028283601044677197933197021484375;3.014660128394303750809513076092116534709930419921875;5.29104737030530003494277480058372020721435546875;1.8018829599315646650126154781901277601718902587890625;-3.780494805335994801254173580673523247241973876953125;-0.82794048304963963058611398082575760781764984130859375;-0.75276220003998017826774002969614230096340179443359375;-0.918260179670823628583775644074194133281707763671875;-1.5960749465646273392849252559244632720947265625;2.280202799305620420255991120939143002033233642578125;0.6798608356003492669827892314060591161251068115234375;0.00037235437068993369746916499707367620430886745452880859375;0.337122632082677398113190747608314268290996551513671875;-1.3454473348402427035352957318536937236785888671875;0.01443955672754803666590905919520082534290850162506103515625;-0.1776195368516353401133756051422096788883209228515625;1.4978387755899638111856120303855277597904205322265625;1.46539531018312541021941797225736081600189208984375;-0.32071205937207902803010028947028331458568572998046875;-1.90744419520537444867613885435275733470916748046875;-11.9891606982089005128955250256694853305816650390625;-2.1669887121737634316787080024369060993194580078125;0.3672127830607030407605861910269595682621002197265625;-0.06203580478551275201315462481943541206419467926025390625;-2.93472369606861160917787856305949389934539794921875;1.75388849018205572605211273184977471828460693359375;0.697291453036331443371409477549605071544647216796875;-0.0645312657524038379985853453035815618932247161865234375;3.764184402430989617727163931704126298427581787109375;1.7961663654062818284984359706868417561054229736328125;-0.8081845398239464461909165038377977907657623291015625;0.78181635523739334558968039345927536487579345703125;-4.5319131193828585679739262559451162815093994140625;0.024789841792795141994787400108180008828639984130859375;-6.117333706507910306982012116350233554840087890625;-1.52321329303906960461745256907306611537933349609375;-0.6842591181818225010147216380573809146881103515625;0.656524530984853083026564490864984691143035888671875;-0.724499291455265481687320061610080301761627197265625;2.936003111628732842319777773809619247913360595703125;-0.87591317415541547486412810030742548406124114990234375;-5.40320016731756869177161206607706844806671142578125;-0.08928640781480877419706843056701472960412502288818359375;2.76745317279060021320447049220092594623565673828125;-0.36100903729607425329817260717391036450862884521484375;-0.2338154075428852951556990547032910399138927459716796875;5.617788840059471766608112375251948833465576171875;-0.18177176297821329153947544909897260367870330810546875;-2.897641100484706466744455610751174390316009521484375 ...(+1531 chars)]
      mask Display: e = 0.06;c1 = [120 150 230]/255;c2 = ([120 150 230]+0)/383;c3 = ([120 150 230]+128)/383;patch([0 1 1 0],[0 0 1 1],c1);patch([0 1 1 1-e 1-e 0+e],[0 0 1 1-e 0+e 0+e],c2);patch([0 0 1 1-e 0+e 0+e],[0 1 1 1-e 1-e 0+e],c3);plot([0 1 1 0 0],[0 0 1 1 0]);disp('b');
  netsum : Sum  Inputs=2  SaturateOnIntegerOverflow=on  InputSameDT=on  OutDataTypeStr=Inherit: Same as first input
      mask Display: e = 0.06;c1 = [120 150 230]/255;c2 = ([120 150 230]+0)/383;c3 = ([120 150 230]+128)/383;patch([0 1 1 0],[0 0 1 1],c1);patch([0 1 1 1-e 1-e 0+e],[0 0 1 1-e 0+e 0+e],c2);patch([0 0 1 1-e 0+e 0+e],[0 1 1 1-e 1-e 0+e],c3);plot([0 1 1 0 0],[0 0 1 1 0]);disp('+');
  tansig : neural/Transfer Functions/tansig
      settings: SourceProductName=Deep Learning Toolbox
  "a{1}" : Outport  InitialOutput=[0;0;0;0;0;0;0;0;0;0;0;0;0;0;0;0;0;0;0;0;0;0;0;0;0;0;0;0;0;0;0;0;0;0;0;0;0;0;0;0;0;0;0;0;0;0;0;0;0;0;0;0;0;0;0;0;0;0;0;0;0;0;0;0;0;0;0;0;0;0;0;0;0;0;0;0;0;0;0;0;0;0;0;0;0;0;0;0;0;0;0;0;0;0;0;0;0;0;0;0]
      mask Display: e = 0.06;c1 = [120 230 180]/255;c2 = ([120 230 180]+0)/(256+128);c3 = ([120 230 180]+128)/(256+128);patch([0 1 1 0],[0 0 1 1],c1);patch([0 1 1 1-e 1-e 0+e],[0 0 1 1-e 0+e 0+e],c2);patch([0 0 1 1-e 0+e 0+e],[0 1 1 1-e 1-e 0+e],c3);plot([0 1 1 0 0],[0 0 1 1 0]);
  wires:
  "p{1}"/1 -> Delays 1/1("p{1}")
  Delays 1/1("pd{1,1}") -> "IW{1,1}"/1("pd{1,1}")
  "IW{1,1}"/1("iz{1,1}") -> netsum/1
  "b{1}"/1 -> netsum/2
  netsum/1 -> tansig/1
  tansig/1 -> "a{1}"/1

== system dynamicANN/BEARING 2 NL/B2NN/Layer 2 ==
  "a{1} " : Inport  PortDimensions=100
      mask Display: e = 0.06;c1 = [120 230 180]/255;c2 = ([120 230 180]+0)/(256+128);c3 = ([120 230 180]+128)/(256+128);patch([0 1 1 0],[0 0 1 1],c1);patch([0 1 1 1-e 1-e 0+e],[0 0 1 1-e 0+e 0+e],c2);patch([0 0 1 1-e 0+e 0+e],[0 1 1 1-e 1-e 0+e],c3);plot([0 1 1 0 0],[0 0 1 1 0]);
  Delays 1 : Subsystem
      mask Display: e = 0.06;c1 = [120 150 230]/255;c2 = ([120 150 230]+0)/383;c3 = ([120 150 230]+128)/383;patch([0 1 1 0],[0 0 1 1],c1);patch([0 1 1 1-e 1-e 0+e],[0 0 1 1-e 0+e 0+e],c2);patch([0 0 1 1-e 0+e 0+e],[0 1 1 1-e 1-e 0+e],c3);plot([0 1 1 0 0],[0 0 1 1 0]);disp('0');
  "LW{2,1}" : Subsystem
      mask Display: e = 0.06;c1 = [120 150 230]/255;c2 = ([120 150 230]+0)/383;c3 = ([120 150 230]+128)/383;patch([0 1 1 0],[0 0 1 1],c1);patch([0 1 1 1-e 1-e 0+e],[0 0 1 1-e 0+e 0+e],c2);patch([0 0 1 1-e 0+e 0+e],[0 1 1 1-e 1-e 0+e],c3);plot([0 1 1 0 0],[0 0 1 1 0]);disp('W');
  "b{2}" : Constant  Value=[0.162145250569083076985776870060362853109836578369140625;3.253717818452451115973644846235401928424835205078125]
      mask Display: e = 0.06;c1 = [120 150 230]/255;c2 = ([120 150 230]+0)/383;c3 = ([120 150 230]+128)/383;patch([0 1 1 0],[0 0 1 1],c1);patch([0 1 1 1-e 1-e 0+e],[0 0 1 1-e 0+e 0+e],c2);patch([0 0 1 1-e 0+e 0+e],[0 1 1 1-e 1-e 0+e],c3);plot([0 1 1 0 0],[0 0 1 1 0]);disp('b');
  netsum : Sum  Inputs=2  SaturateOnIntegerOverflow=on  InputSameDT=on  OutDataTypeStr=Inherit: Same as first input
      mask Display: e = 0.06;c1 = [120 150 230]/255;c2 = ([120 150 230]+0)/383;c3 = ([120 150 230]+128)/383;patch([0 1 1 0],[0 0 1 1],c1);patch([0 1 1 1-e 1-e 0+e],[0 0 1 1-e 0+e 0+e],c2);patch([0 0 1 1-e 0+e 0+e],[0 1 1 1-e 1-e 0+e],c3);plot([0 1 1 0 0],[0 0 1 1 0]);disp('+');
  purelin : neural/Transfer Functions/purelin
      settings: SourceProductName=Deep Learning Toolbox
  "a{2}" : Outport  InitialOutput=[0;0]
      mask Display: e = 0.06;c1 = [120 230 180]/255;c2 = ([120 230 180]+0)/(256+128);c3 = ([120 230 180]+128)/(256+128);patch([0 1 1 0],[0 0 1 1],c1);patch([0 1 1 1-e 1-e 0+e],[0 0 1 1-e 0+e 0+e],c2);patch([0 0 1 1-e 0+e 0+e],[0 1 1 1-e 1-e 0+e],c3);plot([0 1 1 0 0],[0 0 1 1 0]);
  wires:
  "a{1} "/1 -> Delays 1/1("p{2}")
  Delays 1/1("pd{2,1}") -> "LW{2,1}"/1("ad{2,1}")
  "LW{2,1}"/1("lz{2,1}") -> netsum/1
  "b{2}"/1 -> netsum/2
  netsum/1 -> purelin/1
  purelin/1 -> "a{2}"/1

== system dynamicANN/BEARING 2 NL/B2NN/Process Input 1 ==
  x : Inport  PortDimensions=4
      mask Display: e = 0.06;c1 = [120 230 180]/255;c2 = ([120 230 180]+0)/(256+128);c3 = ([120 230 180]+128)/(256+128);patch([0 1 1 0],[0 0 1 1],c1);patch([0 1 1 1-e 1-e 0+e],[0 0 1 1-e 0+e 0+e],c2);patch([0 0 1 1-e 0+e 0+e],[0 1 1 1-e 1-e 0+e],c3);plot([0 1 1 0 0],[0 0 1 1 0]);
  mapminmax : neural/Processing Functions/mapminmax  xmin=[-416.751800229438060796383069828;-77252.7627451588050462305545807;-412.604732780781148449023021385;-87738.2155925167608074843883514]  xmax=[420.767069573879723520803963766;77306.0606816288054687902331352;399.854305951324249690514989197;66574.8201504489697981625795364]  ymin=-1  ymax=1
      settings: SourceProductName=Deep Learning Toolbox
  p : Outport  PortDimensions=4
      mask Display: e = 0.06;c1 = [120 230 180]/255;c2 = ([120 230 180]+0)/(256+128);c3 = ([120 230 180]+128)/(256+128);patch([0 1 1 0],[0 0 1 1],c1);patch([0 1 1 1-e 1-e 0+e],[0 0 1 1-e 0+e 0+e],c2);patch([0 0 1 1-e 0+e 0+e],[0 1 1 1-e 1-e 0+e],c3);plot([0 1 1 0 0],[0 0 1 1 0]);
  wires:
  x/1 -> mapminmax/1
  mapminmax/1 -> p/1

== system dynamicANN/BEARING 2 NL/B2NN/Process Output 1 ==
  a : Inport  PortDimensions=2
      mask Display: e = 0.06;c1 = [120 230 180]/255;c2 = ([120 230 180]+0)/(256+128);c3 = ([120 230 180]+128)/(256+128);patch([0 1 1 0],[0 0 1 1],c1);patch([0 1 1 1-e 1-e 0+e],[0 0 1 1-e 0+e 0+e],c2);patch([0 0 1 1-e 0+e 0+e],[0 1 1 1-e 1-e 0+e],c3);plot([0 1 1 0 0],[0 0 1 1 0]);
  mapminmax_reverse : neural/Processing Functions/mapminmax_reverse  xmin=[-106.274577764110574662481667474;-90.0138039858543947957514319569]  xmax=[105.37554263525613862384489039;121.561184920492564742744434625]  ymin=-1  ymax=1
      settings: SourceProductName=Deep Learning Toolbox
  y : Outport  PortDimensions=2
      mask Display: e = 0.06;c1 = [120 230 180]/255;c2 = ([120 230 180]+0)/(256+128);c3 = ([120 230 180]+128)/(256+128);patch([0 1 1 0],[0 0 1 1],c1);patch([0 1 1 1-e 1-e 0+e],[0 0 1 1-e 0+e 0+e],c2);patch([0 0 1 1-e 0+e 0+e],[0 1 1 1-e 1-e 0+e],c3);plot([0 1 1 0 0],[0 0 1 1 0]);
  wires:
  a/1 -> mapminmax_reverse/1
  mapminmax_reverse/1 -> y/1
